simulink model "DataPath"  (R2025a)
settings: Solver=FixedStepAuto  StartTime=0  StopTime=0.02  FixedStep=1e-7  RelTol=1e-3
undefined symbols (not defined in the file): Bit_1, Bit_2, Bit_3, Bit_4, Bit_5, Bit_6, Bit_7, Bit_8
libraries: simulink_extras x126, fl_lib x34, nesl_utility x18, simulink x2
(part 1 of 7)
settings Model: PacingRate=0.000010  Creator=Erys  LastModifiedBy=Erys
settings DebuggingCC: AlgebraicLoopMsg=none  ForceCombineOutputUpdateInSim=on

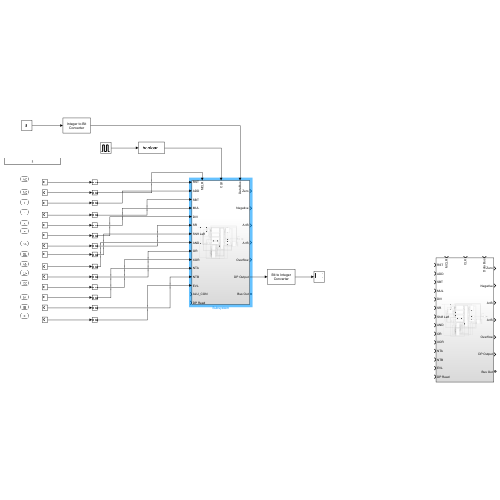
[thumbnail: Simulink's stored preview of the top-level diagram]
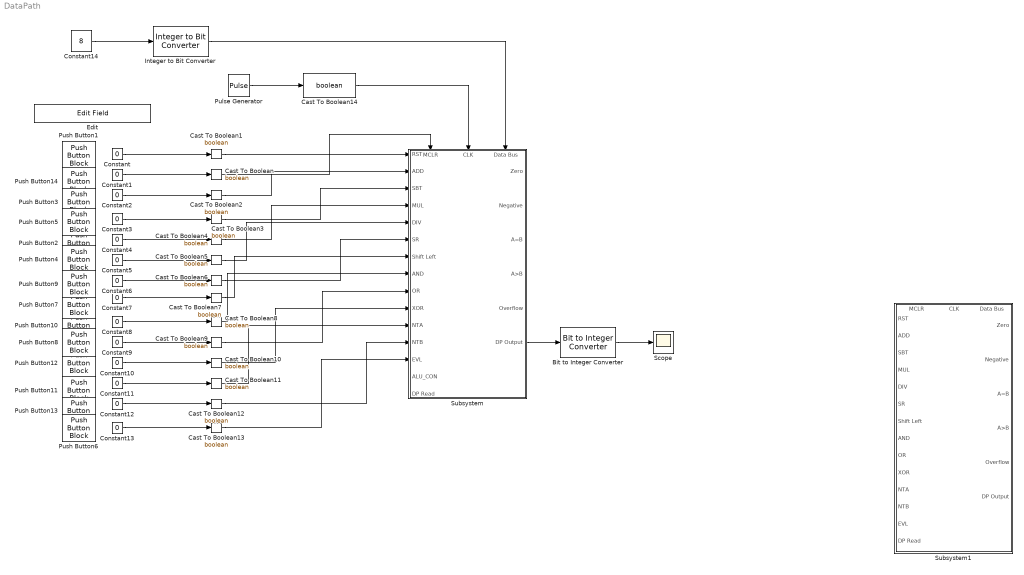
== system DataPath ==
  Bit to Integer Converter : simulink/Logic and Bit Operations/Bit to Integer Converter  nbits=8  bitOrder=MSB first  signedOutputValues=Unsigned  outDtype=Inherit via internal rule  outDtypeSigned=Inherit via internal rule
  Cast To Boolean{,1..14} (15 alike) : DataTypeConversion  OutDataTypeStr=boolean  SaturateOnIntegerOverflow=off  RndMeth=Floor
  Constant{,2..13} (13 alike) : Constant  Value=0
  Constant1 : Constant  Value=0  OutDataTypeStr=boolean
  Constant14 : Constant  Value=8
  Edit : EditField  LabelPosition=Hide  ShowInitialText=on  Alignment=Center
  Integer to Bit Converter : simulink/Logic and Bit Operations/Integer to Bit Converter  nbits=8  signedInputValues=Signed  bitOrder=MSB first  outDtype=Inherit via internal rule
  Pulse Generator : DiscretePulseGenerator  PulseType=Time based  Period=1e-6  PulseWidth=50
  Push Button1 : PushButtonBlock  ButtonText=AC  IconOnColor=[0.0, 0.39215686274509803, 0.0]  IconOffColor=[0.0, 1.0, 0.0]  OffValue=0.000000
  Push Button10 : PushButtonBlock  ButtonText=AND  IconOnColor=[0.0, 0.39215686274509803, 0.0]  IconOffColor=[0.0, 1.0, 0.0]  OffValue=0.000000
  Push Button11 : PushButtonBlock  ButtonText=!A  IconOnColor=[0.0, 0.39215686274509803, 0.0]  IconOffColor=[0.0, 1.0, 0.0]  OffValue=0.000000
  Push Button12 : PushButtonBlock  ButtonText=XOR  IconOnColor=[0.0, 0.39215686274509803, 0.0]  IconOffColor=[0.0, 1.0, 0.0]  OffValue=0.000000
  Push Button13 : PushButtonBlock  ButtonText=!B  IconOnColor=[0.0, 0.39215686274509803, 0.0]  IconOffColor=[0.0, 1.0, 0.0]  OffValue=0.000000
  Push Button14 : PushButtonBlock  ButtonText=MCLR  IconOnColor=[0.0, 0.39215686274509803, 0.0]  IconOffColor=[0.0, 1.0, 0.0]  OffValue=0.000000
  Push Button2 : PushButtonBlock  ButtonText=x  IconOnColor=[0.0, 0.39215686274509803, 0.0]  IconOffColor=[0.0, 1.0, 0.0]  OffValue=0.000000
  Push Button3 : PushButtonBlock  ButtonText=+  IconOnColor=[0.0, 0.39215686274509803, 0.0]  IconOffColor=[0.0, 1.0, 0.0]  OffValue=0.000000
  Push Button4 : PushButtonBlock  ButtonText=÷  IconOnColor=[0.0, 0.39215686274509803, 0.0]  IconOffColor=[0.0, 1.0, 0.0]  OffValue=0.000000
  Push Button5 : PushButtonBlock  ButtonText=-  IconOnColor=[0.0, 0.39215686274509803, 0.0]  IconOffColor=[0.0, 1.0, 0.0]  OffValue=0.000000
  Push Button6 : PushButtonBlock  ButtonText==  IconOnColor=[0.0, 0.39215686274509803, 0.0]  IconOffColor=[0.0, 1.0, 0.0]  OffValue=0.000000
  Push Button7 : PushButtonBlock  ButtonText=SL  IconOnColor=[0.0, 0.39215686274509803, 0.0]  IconOffColor=[0.0, 1.0, 0.0]  OffValue=0.000000
  Push Button8 : PushButtonBlock  ButtonText=OR  IconOnColor=[0.0, 0.39215686274509803, 0.0]  IconOffColor=[0.0, 1.0, 0.0]  OffValue=0.000000
  Push Button9 : PushButtonBlock  ButtonText=SR  IconOnColor=[0.0, 0.39215686274509803, 0.0]  IconOffColor=[0.0, 1.0, 0.0]  OffValue=0.000000
  Scope : Scope
      settings: ActiveDisplayYMinimum=-1.9999999999999996  ActiveDisplayYMaximum=18
  Subsystem : Subsystem
      settings: PortSchema="{\"entries\":[{\"content\":{\"sides\":[{\"content\":{\"connectorIds\":[\"In1\",\"In2\",\"In3\",\"In4\",\"In5\",\"In6\",\"In7\",\"In8\",\"In9\",\"In10\",\"In11\",\"In12\",\"In13\",\"In14\",\"In15\"]},\"type\":\"ConnectorPlacement.EquallySpacedRectSide\",\"uuid\":\"500cbc3b-e28d-47d3-99fc-6c714bf2f9c7\"},{\"content\":{\"connectorIds\":[\"Out1\",\"Out2\",\"Out3\",\"Out4\",\"Out5\",\"Out6\",\"RConn1\"],\"side\":\"RIGHT\"},\"type\":\"ConnectorPlacement.EquallySpacedRectSide\",\"uuid\":\"5d28cb21-17c3-47ed-8e1f-27c0d1cd1a3c\"},{\"content\":{\"connectorIds\":[\"In16\",\"In17\",\"In18\"],\"side\":\"TOP\"},\"type\":\"ConnectorPlacement.EquallySpacedRectSide\",\"uuid\":\"904f1374-4275-4bb1-a3cb-c22725edf960\"},{\"content\":{\"side\":\"BOTTOM\"},\"type\":\"ConnectorPlacement.EquallySpacedRectSide\",\"uuid\":\"1d94aa30-5d0f-4b17-8ccb-c29f6c482f2b\"}]},\"type\":\"ConnectorPlacement.EquallySpacedConnector\",\"uuid\":\"7b6858cb-ce34-402a-a17d-f8242b3d3948\"}],\"packageUris\":[\"http://schema.mathworks.com/mf0/Connector/R2020b\"],\"version\":\"1.0\"}"
  Subsystem1 : Subsystem
      settings: PortSchema="{\"entries\":[{\"content\":{\"sides\":[{\"content\":{\"connectorIds\":[\"In1\",\"In2\",\"In3\",\"In4\",\"In5\",\"In6\",\"In7\",\"In8\",\"In9\",\"In10\",\"In11\",\"In12\",\"In13\",\"In14\"]},\"type\":\"ConnectorPlacement.EquallySpacedRectSide\",\"uuid\":\"500cbc3b-e28d-47d3-99fc-6c714bf2f9c7\"},{\"content\":{\"connectorIds\":[\"Out1\",\"Out2\",\"Out3\",\"Out4\",\"Out5\",\"Out6\",\"RConn1\"],\"side\":\"RIGHT\"},\"type\":\"ConnectorPlacement.EquallySpacedRectSide\",\"uuid\":\"5d28cb21-17c3-47ed-8e1f-27c0d1cd1a3c\"},{\"content\":{\"connectorIds\":[\"In15\",\"In16\",\"In17\"],\"side\":\"TOP\"},\"type\":\"ConnectorPlacement.EquallySpacedRectSide\",\"uuid\":\"904f1374-4275-4bb1-a3cb-c22725edf960\"},{\"content\":{\"side\":\"BOTTOM\"},\"type\":\"ConnectorPlacement.EquallySpacedRectSide\",\"uuid\":\"1d94aa30-5d0f-4b17-8ccb-c29f6c482f2b\"}]},\"type\":\"ConnectorPlacement.EquallySpacedConnector\",\"uuid\":\"7b6858cb-ce34-402a-a17d-f8242b3d3948\"}],\"packageUris\":[\"http://schema.mathworks.com/mf0/Connector/R2020b\"],\"version\":\"1.0\"}"
  wires:
  Constant14/1 -> Integer to Bit Converter/1
  Constant4/1 -> Cast To Boolean4/1
  Constant5/1 -> Cast To Boolean5/1
  Constant3/1 -> Cast To Boolean3/1
  Integer to Bit Converter/1 -> Subsystem/18(Data Bus)
  Constant/1 -> Cast To Boolean1/1
  Constant1/1 -> Cast To Boolean/1
  Constant2/1 -> Cast To Boolean2/1
  Constant6/1 -> Cast To Boolean6/1
  Constant7/1 -> Cast To Boolean7/1
  Constant8/1 -> Cast To Boolean8/1
  Constant9/1 -> Cast To Boolean9/1
  Constant10/1 -> Cast To Boolean10/1
  Constant11/1 -> Cast To Boolean11/1
  Constant12/1 -> Cast To Boolean12/1
  Constant13/1 -> Cast To Boolean13/1
  Pulse Generator/1 -> Cast To Boolean14/1
  Cast To Boolean1/1 -> Subsystem/1(RST)
  Cast To Boolean/1 -> Subsystem/16(MCLR)
  Cast To Boolean2/1 -> Subsystem/2(ADD)
  Cast To Boolean3/1 -> Subsystem/3(SBT)
  Cast To Boolean4/1 -> Subsystem/4(MUL)
  Cast To Boolean5/1 -> Subsystem/5(DIV)
  Cast To Boolean6/1 -> Subsystem/6(SR)
  Cast To Boolean7/1 -> Subsystem/7(Shift Left)
  Cast To Boolean8/1 -> Subsystem/8(AND)
  Cast To Boolean9/1 -> Subsystem/9(OR)
  Cast To Boolean10/1 -> Subsystem/10(XOR)
  Cast To Boolean11/1 -> Subsystem/11(NTA)
  Cast To Boolean12/1 -> Subsystem/12(NTB)
  Cast To Boolean13/1 -> Subsystem/13(EVL)
  Subsystem/6(DP Output) -> Bit to Integer Converter/1
  Bit to Integer Converter/1 -> Scope/1
  Cast To Boolean14/1 -> Subsystem/17(CLK)

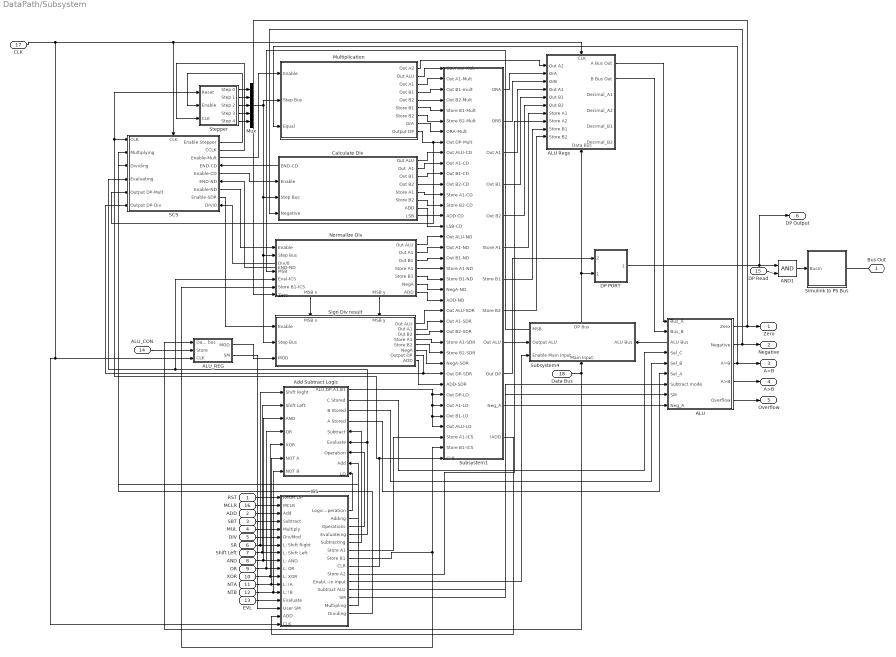
== system DataPath/Subsystem ==
  RST : Inport
  ADD : Inport  Port=2
  SBT : Inport  Port=3
  MUL : Inport  Port=4
  DIV : Inport  Port=5
  SR : Inport  Port=6
  Shift Left : Inport  Port=7
  AND : Inport  Port=8
  OR : Inport  Port=9
  XOR : Inport  Port=10
  NTA : Inport  Port=11
  NTB : Inport  Port=12
  EVL : Inport  Port=13
  ALU_CON : Inport  Port=14
  DP Read : Inport  Port=15
  MCLR : Inport  Port=16  OutDataTypeStr=boolean
  CLK : Inport  Port=17  OutDataTypeStr=boolean
  Data Bus : Inport  Port=18
  ALU : Subsystem
      settings: PortSchema="{\"entries\":[{\"content\":{\"sides\":[{\"content\":{\"connectorIds\":[\"In1\",\"In2\",\"Out6\",\"In3\",\"In4\",\"In5\",\"In6\",\"In7\",\"In8\"]},\"type\":\"ConnectorPlacement.EquallySpacedRectSide\",\"uuid\":\"c37a7539-9d16-4848-9066-29ecf491d7da\"},{\"content\":{\"connectorIds\":[\"Out1\",\"Out2\",\"Out3\",\"Out4\",\"Out5\"],\"side\":\"RIGHT\"},\"type\":\"ConnectorPlacement.EquallySpacedRectSide\",\"uuid\":\"a0e4cd93-9d4f-4763-9532-ee9322d920da\"},{\"content\":{\"side\":\"TOP\"},\"type\":\"ConnectorPlacement.EquallySpacedRectSide\",\"uuid\":\"186aeace-b60a-4a73-952e-f0bee95a6888\"}]},\"type\":\"ConnectorPlacement.EquallySpacedConnector\",\"uuid\":\"47b774ea-3904-45d1-ac98-1d3dfdc91dee\"}],\"packageUris\":[\"http://schema.mathworks.com/mf0/Connector/R2020b\"],\"version\":\"1.0\"}"
  ALU Regs : Subsystem
      settings: PortSchema="{\"entries\":[{\"content\":{\"sides\":[{\"content\":{\"connectorIds\":[\"In1\",\"In2\",\"In3\",\"In4\",\"In5\",\"In6\",\"In7\",\"In8\",\"In9\",\"In10\"]},\"type\":\"ConnectorPlacement.EquallySpacedRectSide\",\"uuid\":\"f897ceb0-c9b9-489e-8b32-2eb573f12d1a\"},{\"content\":{\"connectorIds\":[\"Out1\",\"Out2\",\"Out3\",\"Out4\",\"Out5\",\"Out6\"],\"side\":\"RIGHT\"},\"type\":\"ConnectorPlacement.EquallySpacedRectSide\",\"uuid\":\"50fe41fa-7ee3-4a8d-a06d-fa2133f944ed\"},{\"content\":{\"connectorIds\":[\"In11\"],\"side\":\"TOP\"},\"type\":\"ConnectorPlacement.EquallySpacedRectSide\",\"uuid\":\"9386cea2-fe71-481a-887c-1138907670aa\"},{\"content\":{\"connectorIds\":[\"In12\"],\"side\":\"BOTTOM\"},\"type\":\"ConnectorPlacement.EquallySpacedRectSide\",\"uuid\":\"2c9e15c6-049a-46aa-8a1e-0778ad228e2c\"}]},\"type\":\"ConnectorPlacement.EquallySpacedConnector\",\"uuid\":\"51e3a67b-2c64-426e-a2d7-da64166e8617\"}],\"packageUris\":[\"http://schema.mathworks.com/mf0/Connector/R2020b\"],\"version\":\"1.0\"}"
  ALU_REG : Subsystem
  AND1 : Logic  IconShape=distinctive  AllPortsSameDT=off  OutDataTypeStr=boolean
  Add Subtract Logic : Subsystem
      settings: PortSchema="{\"entries\":[{\"content\":{\"sides\":[{\"content\":{\"connectorIds\":[\"In1\",\"In2\",\"In3\",\"In4\",\"In5\",\"In6\",\"In7\"]},\"type\":\"ConnectorPlacement.EquallySpacedRectSide\",\"uuid\":\"155e8539-7b07-4c7c-9d9a-97cd4ac10054\"},{\"content\":{\"connectorIds\":[\"Out1\",\"Out2\",\"Out3\",\"Out4\",\"In8\",\"In9\",\"In10\",\"In11\",\"In12\"],\"side\":\"RIGHT\"},\"type\":\"ConnectorPlacement.EquallySpacedRectSide\",\"uuid\":\"e444004c-3fa4-46de-94bb-9c3dc8287e68\"},{\"content\":{\"side\":\"TOP\"},\"type\":\"ConnectorPlacement.EquallySpacedRectSide\",\"uuid\":\"07fd3642-a6d7-4398-b7f9-f213a05a7aff\"}]},\"type\":\"ConnectorPlacement.EquallySpacedConnector\",\"uuid\":\"401fffe2-fef7-4730-8c52-e9531038c85b\"}],\"packageUris\":[\"http://schema.mathworks.com/mf0/Connector/R2020b\"],\"version\":\"1.0\"}"
  Calculate Div : Subsystem
      settings: PortSchema="{\"entries\":[{\"content\":{\"sides\":[{\"content\":{\"connectorIds\":[\"Out9\",\"In1\",\"In2\",\"In3\"]},\"type\":\"ConnectorPlacement.EquallySpacedRectSide\",\"uuid\":\"248e61db-650f-41be-afeb-960a1b0fa547\"},{\"content\":{\"connectorIds\":[\"Out1\",\"Out2\",\"Out3\",\"Out4\",\"Out5\",\"Out6\",\"Out7\",\"Out8\"],\"side\":\"RIGHT\"},\"type\":\"ConnectorPlacement.EquallySpacedRectSide\",\"uuid\":\"a5a9d453-5aa0-49ce-8cbc-1e6a6fbe953d\"},{\"content\":{\"side\":\"TOP\"},\"type\":\"ConnectorPlacement.EquallySpacedRectSide\",\"uuid\":\"161ea693-d847-495c-b99e-fc66d877945e\"}]},\"type\":\"ConnectorPlacement.EquallySpacedConnector\",\"uuid\":\"e6ca75ed-542b-4a47-8d6b-6b616e1ea101\"}],\"packageUris\":[\"http://schema.mathworks.com/mf0/Connector/R2020b\"],\"version\":\"1.0\"}"
  DP PORT : Subsystem
  ICS : Subsystem
  Multiplication : Subsystem
  Mux : Mux  Inputs=5
  Normalize Div : Subsystem
      settings: PortSchema="{\"entries\":[{\"content\":{\"sides\":[{\"content\":{\"connectorIds\":[\"Out10\",\"In1\",\"In2\",\"Out11\",\"In3\",\"In4\",\"In5\",\"In6\"]},\"type\":\"ConnectorPlacement.EquallySpacedRectSide\",\"uuid\":\"3bf65de4-a84e-43af-85cb-ba419936807e\"},{\"content\":{\"connectorIds\":[\"Out1\",\"Out2\",\"Out3\",\"Out4\",\"Out5\",\"Out6\",\"Out7\"],\"side\":\"RIGHT\"},\"type\":\"ConnectorPlacement.EquallySpacedRectSide\",\"uuid\":\"49151b5f-73cb-49db-8fd7-1652ca273db5\"},{\"content\":{\"side\":\"TOP\"},\"type\":\"ConnectorPlacement.EquallySpacedRectSide\",\"uuid\":\"58143683-5a5d-47e2-b921-db5f028b3f5b\"},{\"content\":{\"connectorIds\":[\"Out8\",\"Out9\"],\"side\":\"BOTTOM\"},\"type\":\"ConnectorPlacement.EquallySpacedRectSide\",\"uuid\":\"3e5cf15a-3bf5-42b9-8752-baa0123e7179\"}]},\"type\":\"ConnectorPlacement.EquallySpacedConnector\",\"uuid\":\"daef8ab5-bc49-4af8-b635-2b796b1e5932\"}],\"packageUris\":[\"http://schema.mathworks.com/mf0/Connector/R2020b\"],\"version\":\"1.0\"}"
  SCS : Subsystem
      settings: PortSchema="{\"entries\":[{\"content\":{\"sides\":[{\"content\":{\"connectorIds\":[\"In1\",\"In2\",\"In3\",\"In4\",\"In5\",\"In6\"]},\"type\":\"ConnectorPlacement.EquallySpacedRectSide\",\"uuid\":\"5f827d29-1953-485f-9672-5b30f3e9777e\"},{\"content\":{\"connectorIds\":[\"Out1\",\"Out2\",\"Out3\",\"In8\",\"Out4\",\"In9\",\"Out5\",\"Out6\",\"In10\"],\"side\":\"RIGHT\"},\"type\":\"ConnectorPlacement.EquallySpacedRectSide\",\"uuid\":\"f4b83631-e908-4486-8992-7d28022d8f8a\"},{\"content\":{\"connectorIds\":[\"In7\"],\"side\":\"TOP\"},\"type\":\"ConnectorPlacement.EquallySpacedRectSide\",\"uuid\":\"92fa476f-0825-43c4-abf8-7a9cce9eadb6\"}]},\"type\":\"ConnectorPlacement.EquallySpacedConnector\",\"uuid\":\"7f47888f-0f87-43c3-bf1c-119855c5fec8\"}],\"packageUris\":[\"http://schema.mathworks.com/mf0/Connector/R2020b\"],\"version\":\"1.0\"}"
  Sign Div result : Subsystem
      settings: PortSchema="{\"entries\":[{\"content\":{\"sides\":[{\"content\":{\"connectorIds\":[\"In1\",\"In2\",\"In3\"]},\"type\":\"ConnectorPlacement.EquallySpacedRectSide\",\"uuid\":\"f5bc0604-c60b-487e-b7f2-96d42dc1b3a0\"},{\"content\":{\"connectorIds\":[\"Out1\",\"Out2\",\"Out3\",\"Out4\",\"Out5\",\"Out6\",\"Out7\",\"Out8\"],\"side\":\"RIGHT\"},\"type\":\"ConnectorPlacement.EquallySpacedRectSide\",\"uuid\":\"50d41b4c-a33b-4e34-b751-18ded5b2cb1e\"},{\"content\":{\"connectorIds\":[\"In4\",\"In5\"],\"side\":\"TOP\"},\"type\":\"ConnectorPlacement.EquallySpacedRectSide\",\"uuid\":\"1ba562d7-8709-4333-a841-74571fdc4e92\"}]},\"type\":\"ConnectorPlacement.EquallySpacedConnector\",\"uuid\":\"8253a047-369e-44b5-9bb6-13f033f299b7\"}],\"packageUris\":[\"http://schema.mathworks.com/mf0/Connector/R2020b\"],\"version\":\"1.0\"}"
  Simulink to PS Bus : Subsystem
  Stepper : Subsystem
  Subsystem1 : Subsystem
  Subsystem4 : Subsystem
      settings: PortSchema="{\"entries\":[{\"content\":{\"sides\":[{\"content\":{\"connectorIds\":[\"Out2\"]},\"type\":\"ConnectorPlacement.EquallySpacedRectSide\",\"uuid\":\"d8595652-6905-4cc2-aa18-713ce57c3b65\"},{\"content\":{\"connectorIds\":[\"In4\"],\"side\":\"RIGHT\"},\"type\":\"ConnectorPlacement.EquallySpacedRectSide\",\"uuid\":\"5abc3ebd-ff8c-460a-ade3-5894559f8820\"},{\"content\":{\"connectorIds\":[\"Out1\",\"In1\",\"In2\"],\"side\":\"TOP\"},\"type\":\"ConnectorPlacement.EquallySpacedRectSide\",\"uuid\":\"929f6aeb-a855-409a-8e7c-28fb07fb21dc\"},{\"content\":{\"connectorIds\":[\"In3\"],\"side\":\"BOTTOM\"},\"type\":\"ConnectorPlacement.EquallySpacedRectSide\",\"uuid\":\"480c7dc4-4298-475d-8e28-71ecbd723b86\"}]},\"type\":\"ConnectorPlacement.EquallySpacedConnector\",\"uuid\":\"31897c44-8fce-467c-9d36-164830a373ff\"}],\"packageUris\":[\"http://schema.mathworks.com/mf0/Connector/R2020b\"],\"version\":\"1.0\"}"
  Bus Out : PMIOPort  Side=Right
  Zero : Outport
  Negative : Outport  Port=2
  A=B : Outport  Port=3
  A>B : Outport  Port=4
  Overflow : Outport  Port=5
  DP Output : Outport  Port=6
  wires:
  Stepper/1(Step 0) -> Mux/1
  Stepper/2(Step 1) -> Mux/2
  Stepper/5(Step 4) -> Mux/5
  Stepper/4(Step 3) -> Mux/4
  Stepper/3(Step 2) -> Mux/3
  Normalize Div/8(MSB x) -> Sign Div result/4(MSB x)
  Normalize Div/9(MSB y) -> Sign Div result/5(MSB y)
  Multiplication/2(Out ALU) -> Subsystem1/1(Out ALU-Mult)
  Multiplication/3(Out A1) -> Subsystem1/2(Out A1-Mult)
  Multiplication/4(Out B1) -> Subsystem1/3(Out B1-mult)
  Multiplication/5(Out B2) -> Subsystem1/4(Out B2-Mult)
  Multiplication/6(Store B1) -> Subsystem1/5(Store B1-Mult)
  Multiplication/7(Store B2) -> Subsystem1/6(Store B2-Mult)
  Multiplication/8(OrA) -> Subsystem1/7(ORA-Mult)
  Multiplication/9(Output DP) -> SCS/5(Output DP-Mult), Subsystem1/8(Out DP-Mult)
  Calculate Div/1(Out ALU) -> Subsystem1/9(Out ALU-CD)
  Calculate Div/2(Out  A1) -> Subsystem1/10(Out A1-CD)
  Calculate Div/5(Store A1) -> Subsystem1/13(Store A1-CD)
  Calculate Div/6(Store B2) -> Subsystem1/14(Store B2-CD)
  Calculate Div/7(ADD) -> Subsystem1/15(ADD CD)
  Calculate Div/8(LSB) -> Subsystem1/16(LSB-CD)
  Normalize Div/1(Out ALU) -> Subsystem1/17(Out ALU-ND)
  Normalize Div/2(Out A1) -> Subsystem1/18(Out A1-ND)
  Normalize Div/3(Out B1) -> Subsystem1/19(Out B1-ND)
  Normalize Div/4(Store A1) -> Subsystem1/20(Store A1-ND)
  Normalize Div/5(Store B1) -> Subsystem1/21(Store B1-ND)
  Normalize Div/6(NegA) -> Subsystem1/22(NegA-ND)
  Normalize Div/7(ADD) -> Subsystem1/23(ADD-ND)
  Sign Div result/1(Out ALU) -> Subsystem1/24(Out ALU-SDR)
  Sign Div result/2(Out A1) -> Subsystem1/25(Out A1-SDR)
  Sign Div result/3(Out B2) -> Subsystem1/26(Out B2-SDR)
  Sign Div result/4(Store A1) -> Subsystem1/27(Store A1-SDR)
  Sign Div result/5(Store B2) -> Subsystem1/28(Store B2-SDR)
  Sign Div result/6(NegA) -> Subsystem1/29(NegA-SDR)
  Sign Div result/7(Output DP) -> SCS/6(Output DP-Div), Subsystem1/30(Out DP-SDR)
  Add Subtract Logic/1(ALU,DP,A1,B1) -> Subsystem1/32(Out DP-LO), Subsystem1/33(Out A1-LO), Subsystem1/34(Out B1-LO), Subsystem1/35(Out ALU-LO)
  ICS/6(Store A1) -> Subsystem1/36(Store A1-ICS)
  ICS/7(Store B1) -> Subsystem1/37(Store B1-ICS), Normalize Div/5(Store B1-ICS)
  ICS/8(CLR) -> Subsystem1/38(CLR), SCS/1(CLR), Stepper/1(Reset)
  SCS/3(Enable-Mult) -> Multiplication/1(Enable)
  Calculate Div/9(END-CD) -> SCS/8(END-CD)
  SCS/4(Enable-CD) -> Calculate Div/1(Enable)
  Normalize Div/10(END-ND) -> SCS/9(END-ND)
  SCS/5(Enable-ND) -> Normalize Div/1(Enable)
  SCS/6(Enable-SDR) -> Sign Div result/1(Enable)
  Mux/1 -> Calculate Div/2(Step Bus), Sign Div result/2(Step Bus), Normalize Div/2(Step Bus), Multiplication/2(Step Bus)
  SCS/1(Enable Stepper) -> Stepper/2(Enable)
  SCS/2(CCLK) -> Stepper/3(CLK)
  Normalize Div/11(Div/0) -> SCS/10(DIV/0)
  ICS/10(Enable main input) -> Subsystem4/2(Enable Main Input)
  Subsystem1/9(Out ALU) -> Subsystem4/1(Output ALU)
  Subsystem1/10(Out DP) -> DP PORT/2(Enable)
  ALU/6(ALU Bus) -> Subsystem4/3(ALU Bus)
  Subsystem4/2(DP Bus) -> ALU Regs/12(Data Bus), DP PORT/1(DP Bus)
  Subsystem1/3(Out A1) -> ALU Regs/4(Out A1)
  Subsystem1/4(Out B1) -> ALU Regs/5(Out B1)
  Subsystem1/5(Out B2) -> ALU Regs/6(Out B2)
  Subsystem1/6(Store A1) -> ALU Regs/7(Store A1)
  Subsystem1/8(Store B2) -> ALU Regs/10(Store B2)
  Subsystem1/11(Neg_A) -> ALU/8(Neg_A)
  Multiplication/1(Out A2) -> ALU Regs/1(Out A2)
  Add Subtract Logic/2(C Stored) -> ALU/3(Sel_C)
  Add Subtract Logic/3(B Stored) -> ALU/4(Sel_B)
  Add Subtract Logic/4(A Stored) -> ALU/5(Sel_A)
  ALU Regs/1(A Bus Out) -> ALU/1(Bus_A)
  ALU Regs/2(B Bus Out) -> ALU/2(Bus_B)
  ICS/9(Store A2) -> ALU Regs/8(Store A2)
  Subsystem1/7(Store B1) -> ALU Regs/9(Store B1)
  ALU/2(Negative) -> Negative/1, Calculate Div/3(Negative)
  ALU/1(Zero) -> Zero/1, Normalize Div/6(Zero)
  ALU/3(A=B) -> A=B/1, Multiplication/3(Equal)
  ALU/4(A>B) -> A>B/1
  RST/1 -> ICS/1(Reset DP)
  MCLR/1 -> ICS/2(MCLR)
  ADD/1 -> ICS/3(Add)
  SBT/1 -> ICS/4(Subtract)
  MUL/1 -> ICS/5(Multiply)
  DIV/1 -> ICS/6(Div/Mod)
  SR/1 -> Add Subtract Logic/1(Shift Right), ICS/7(L: Shift Right)
  Shift Left/1 -> Add Subtract Logic/2(Shift Left), ICS/8(L: Shift Left)
  AND/1 -> ICS/9(L: AND), Add Subtract Logic/3(AND)
  OR/1 -> Add Subtract Logic/4(OR), ICS/10(L: OR)
  XOR/1 -> Add Subtract Logic/5(XOR), ICS/11(L: XOR)
  NTA/1 -> Add Subtract Logic/6(NOT A), ICS/12(L: !A)
  NTB/1 -> Add Subtract Logic/7(NOT B), ICS/13(L: !B)
  EVL/1 -> ICS/14(Evaluate)
  ALU_REG/2(SM) -> ICS/15(User SM)
  Subsystem1/12("!ADD ") -> ICS/16(ADD)
  ICS/1(Logic Operation) -> Add Subtract Logic/12(LO)
  ICS/2(Adding) -> Add Subtract Logic/11(Add)
  ICS/3(Operations) -> Add Subtract Logic/10(Operation)
  ICS/4(Evaluateing) -> Add Subtract Logic/9(Evaluate), SCS/4(Evaluating), Normalize Div/4(Eval-ICS)
  ICS/5(Subtracting) -> Add Subtract Logic/8(Subtract)
  ICS/11(Subtract ALU) -> ALU/6(Subtract mode)
  ICS/12(SM) -> ALU/7(SM)
  ICS/13(Multipling) -> SCS/2(Multiplying)
  ICS/14(Dividing) -> SCS/3(Dividing)
  CLK/1 -> SCS/7(CLK), ALU Regs/11(CLK), ALU_REG/3(CLK), ICS/17(CLK)
  ALU_CON/1 -> ALU_REG/2(Store)
  DP PORT/1(DP Output) -> DP Output/1, AND1/1
  Subsystem4/1(MSB) -> Normalize Div/3(MSB)
  Data Bus/1 -> Subsystem4/4(Main Input), ALU_REG/1(Data bus)
  Subsystem1/1(ORA) -> ALU Regs/2(OrA)
  Subsystem1/2(ORB) -> ALU Regs/3(OrB)
  Calculate Div/3(Out B1) -> Subsystem1/11(Out B1-CD)
  Calculate Div/4(Out B2) -> Subsystem1/12(Out B2-CD)
  Sign Div result/8(ADD) -> Subsystem1/31(ADD-SDR)
  ALU/5(Overflow) -> Overflow/1
  ALU_REG/1(MOD) -> Sign Div result/3(MOD)
  AND1/1 -> Simulink to PS Bus/1(BusIn)
  DP Read/1 -> AND1/2
  connections:
  Bus Out/RConn1 -- Simulink to PS Bus/RConn1

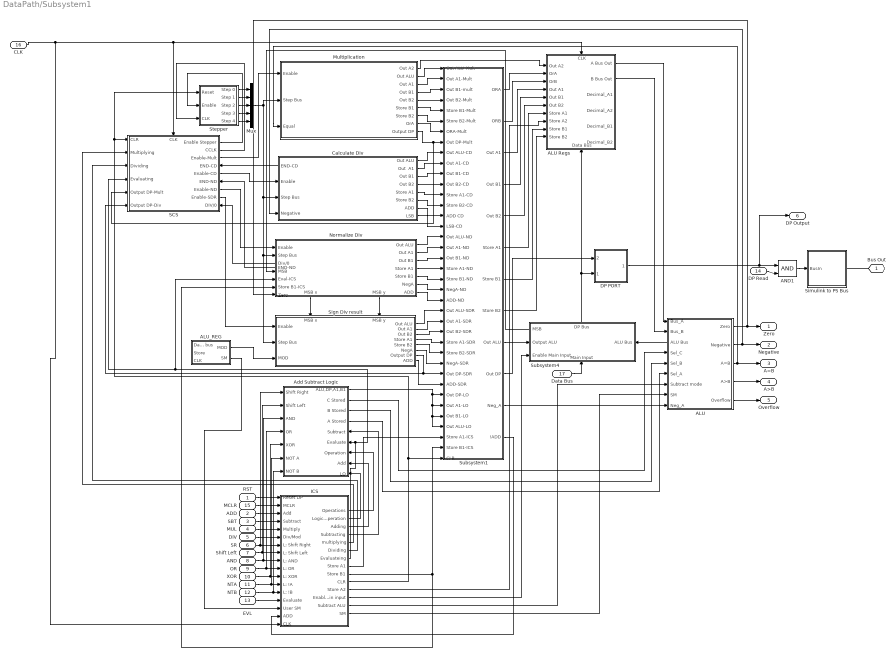
== system DataPath/Subsystem1 ==
  RST : Inport
  ADD : Inport  Port=2
  SBT : Inport  Port=3
  MUL : Inport  Port=4
  DIV : Inport  Port=5
  SR : Inport  Port=6
  Shift Left : Inport  Port=7
  AND : Inport  Port=8
  OR : Inport  Port=9
  XOR : Inport  Port=10
  NTA : Inport  Port=11
  NTB : Inport  Port=12
  EVL : Inport  Port=13
  DP Read : Inport  Port=14
  MCLR : Inport  Port=15  OutDataTypeStr=boolean
  CLK : Inport  Port=16  OutDataTypeStr=boolean
  Data Bus : Inport  Port=17
  ALU : Subsystem
      settings: PortSchema="{\"entries\":[{\"content\":{\"sides\":[{\"content\":{\"connectorIds\":[\"In1\",\"In2\",\"Out6\",\"In3\",\"In4\",\"In5\",\"In6\",\"In7\",\"In8\"]},\"type\":\"ConnectorPlacement.EquallySpacedRectSide\",\"uuid\":\"c37a7539-9d16-4848-9066-29ecf491d7da\"},{\"content\":{\"connectorIds\":[\"Out1\",\"Out2\",\"Out3\",\"Out4\",\"Out5\"],\"side\":\"RIGHT\"},\"type\":\"ConnectorPlacement.EquallySpacedRectSide\",\"uuid\":\"a0e4cd93-9d4f-4763-9532-ee9322d920da\"},{\"content\":{\"side\":\"TOP\"},\"type\":\"ConnectorPlacement.EquallySpacedRectSide\",\"uuid\":\"186aeace-b60a-4a73-952e-f0bee95a6888\"}]},\"type\":\"ConnectorPlacement.EquallySpacedConnector\",\"uuid\":\"47b774ea-3904-45d1-ac98-1d3dfdc91dee\"}],\"packageUris\":[\"http://schema.mathworks.com/mf0/Connector/R2020b\"],\"version\":\"1.0\"}"
  ALU Regs : Subsystem
      settings: PortSchema="{\"entries\":[{\"content\":{\"sides\":[{\"content\":{\"connectorIds\":[\"In1\",\"In2\",\"In3\",\"In4\",\"In5\",\"In6\",\"In7\",\"In8\",\"In9\",\"In10\"]},\"type\":\"ConnectorPlacement.EquallySpacedRectSide\",\"uuid\":\"f897ceb0-c9b9-489e-8b32-2eb573f12d1a\"},{\"content\":{\"connectorIds\":[\"Out1\",\"Out2\",\"Out3\",\"Out4\",\"Out5\",\"Out6\"],\"side\":\"RIGHT\"},\"type\":\"ConnectorPlacement.EquallySpacedRectSide\",\"uuid\":\"50fe41fa-7ee3-4a8d-a06d-fa2133f944ed\"},{\"content\":{\"connectorIds\":[\"In11\"],\"side\":\"TOP\"},\"type\":\"ConnectorPlacement.EquallySpacedRectSide\",\"uuid\":\"9386cea2-fe71-481a-887c-1138907670aa\"},{\"content\":{\"connectorIds\":[\"In12\"],\"side\":\"BOTTOM\"},\"type\":\"ConnectorPlacement.EquallySpacedRectSide\",\"uuid\":\"2c9e15c6-049a-46aa-8a1e-0778ad228e2c\"}]},\"type\":\"ConnectorPlacement.EquallySpacedConnector\",\"uuid\":\"51e3a67b-2c64-426e-a2d7-da64166e8617\"}],\"packageUris\":[\"http://schema.mathworks.com/mf0/Connector/R2020b\"],\"version\":\"1.0\"}"
  ALU_REG : Subsystem
  AND1 : Logic  IconShape=distinctive  AllPortsSameDT=off  OutDataTypeStr=boolean
  Add Subtract Logic : Subsystem
      settings: PortSchema="{\"entries\":[{\"content\":{\"sides\":[{\"content\":{\"connectorIds\":[\"In1\",\"In2\",\"In3\",\"In4\",\"In5\",\"In6\",\"In7\"]},\"type\":\"ConnectorPlacement.EquallySpacedRectSide\",\"uuid\":\"155e8539-7b07-4c7c-9d9a-97cd4ac10054\"},{\"content\":{\"connectorIds\":[\"Out1\",\"Out2\",\"Out3\",\"Out4\",\"In8\",\"In9\",\"In10\",\"In11\",\"In12\"],\"side\":\"RIGHT\"},\"type\":\"ConnectorPlacement.EquallySpacedRectSide\",\"uuid\":\"e444004c-3fa4-46de-94bb-9c3dc8287e68\"},{\"content\":{\"side\":\"TOP\"},\"type\":\"ConnectorPlacement.EquallySpacedRectSide\",\"uuid\":\"07fd3642-a6d7-4398-b7f9-f213a05a7aff\"}]},\"type\":\"ConnectorPlacement.EquallySpacedConnector\",\"uuid\":\"401fffe2-fef7-4730-8c52-e9531038c85b\"}],\"packageUris\":[\"http://schema.mathworks.com/mf0/Connector/R2020b\"],\"version\":\"1.0\"}"
  Calculate Div : Subsystem
      settings: PortSchema="{\"entries\":[{\"content\":{\"sides\":[{\"content\":{\"connectorIds\":[\"Out9\",\"In1\",\"In2\",\"In3\"]},\"type\":\"ConnectorPlacement.EquallySpacedRectSide\",\"uuid\":\"248e61db-650f-41be-afeb-960a1b0fa547\"},{\"content\":{\"connectorIds\":[\"Out1\",\"Out2\",\"Out3\",\"Out4\",\"Out5\",\"Out6\",\"Out7\",\"Out8\"],\"side\":\"RIGHT\"},\"type\":\"ConnectorPlacement.EquallySpacedRectSide\",\"uuid\":\"a5a9d453-5aa0-49ce-8cbc-1e6a6fbe953d\"},{\"content\":{\"side\":\"TOP\"},\"type\":\"ConnectorPlacement.EquallySpacedRectSide\",\"uuid\":\"161ea693-d847-495c-b99e-fc66d877945e\"}]},\"type\":\"ConnectorPlacement.EquallySpacedConnector\",\"uuid\":\"e6ca75ed-542b-4a47-8d6b-6b616e1ea101\"}],\"packageUris\":[\"http://schema.mathworks.com/mf0/Connector/R2020b\"],\"version\":\"1.0\"}"
  DP PORT : Subsystem
  ICS : Subsystem
  Multiplication : Subsystem
  Mux : Mux  Inputs=5
  Normalize Div : Subsystem
      settings: PortSchema="{\"entries\":[{\"content\":{\"sides\":[{\"content\":{\"connectorIds\":[\"Out10\",\"In1\",\"In2\",\"Out11\",\"In3\",\"In4\",\"In5\",\"In6\"]},\"type\":\"ConnectorPlacement.EquallySpacedRectSide\",\"uuid\":\"3bf65de4-a84e-43af-85cb-ba419936807e\"},{\"content\":{\"connectorIds\":[\"Out1\",\"Out2\",\"Out3\",\"Out4\",\"Out5\",\"Out6\",\"Out7\"],\"side\":\"RIGHT\"},\"type\":\"ConnectorPlacement.EquallySpacedRectSide\",\"uuid\":\"49151b5f-73cb-49db-8fd7-1652ca273db5\"},{\"content\":{\"side\":\"TOP\"},\"type\":\"ConnectorPlacement.EquallySpacedRectSide\",\"uuid\":\"58143683-5a5d-47e2-b921-db5f028b3f5b\"},{\"content\":{\"connectorIds\":[\"Out8\",\"Out9\"],\"side\":\"BOTTOM\"},\"type\":\"ConnectorPlacement.EquallySpacedRectSide\",\"uuid\":\"3e5cf15a-3bf5-42b9-8752-baa0123e7179\"}]},\"type\":\"ConnectorPlacement.EquallySpacedConnector\",\"uuid\":\"daef8ab5-bc49-4af8-b635-2b796b1e5932\"}],\"packageUris\":[\"http://schema.mathworks.com/mf0/Connector/R2020b\"],\"version\":\"1.0\"}"
  SCS : Subsystem
      settings: PortSchema="{\"entries\":[{\"content\":{\"sides\":[{\"content\":{\"connectorIds\":[\"In1\",\"In2\",\"In3\",\"In4\",\"In5\",\"In6\"]},\"type\":\"ConnectorPlacement.EquallySpacedRectSide\",\"uuid\":\"5f827d29-1953-485f-9672-5b30f3e9777e\"},{\"content\":{\"connectorIds\":[\"Out1\",\"Out2\",\"Out3\",\"In8\",\"Out4\",\"In9\",\"Out5\",\"Out6\",\"In10\"],\"side\":\"RIGHT\"},\"type\":\"ConnectorPlacement.EquallySpacedRectSide\",\"uuid\":\"f4b83631-e908-4486-8992-7d28022d8f8a\"},{\"content\":{\"connectorIds\":[\"In7\"],\"side\":\"TOP\"},\"type\":\"ConnectorPlacement.EquallySpacedRectSide\",\"uuid\":\"92fa476f-0825-43c4-abf8-7a9cce9eadb6\"}]},\"type\":\"ConnectorPlacement.EquallySpacedConnector\",\"uuid\":\"7f47888f-0f87-43c3-bf1c-119855c5fec8\"}],\"packageUris\":[\"http://schema.mathworks.com/mf0/Connector/R2020b\"],\"version\":\"1.0\"}"
  Sign Div result : Subsystem
      settings: PortSchema="{\"entries\":[{\"content\":{\"sides\":[{\"content\":{\"connectorIds\":[\"In1\",\"In2\",\"In3\"]},\"type\":\"ConnectorPlacement.EquallySpacedRectSide\",\"uuid\":\"f5bc0604-c60b-487e-b7f2-96d42dc1b3a0\"},{\"content\":{\"connectorIds\":[\"Out1\",\"Out2\",\"Out3\",\"Out4\",\"Out5\",\"Out6\",\"Out7\",\"Out8\"],\"side\":\"RIGHT\"},\"type\":\"ConnectorPlacement.EquallySpacedRectSide\",\"uuid\":\"50d41b4c-a33b-4e34-b751-18ded5b2cb1e\"},{\"content\":{\"connectorIds\":[\"In4\",\"In5\"],\"side\":\"TOP\"},\"type\":\"ConnectorPlacement.EquallySpacedRectSide\",\"uuid\":\"1ba562d7-8709-4333-a841-74571fdc4e92\"}]},\"type\":\"ConnectorPlacement.EquallySpacedConnector\",\"uuid\":\"8253a047-369e-44b5-9bb6-13f033f299b7\"}],\"packageUris\":[\"http://schema.mathworks.com/mf0/Connector/R2020b\"],\"version\":\"1.0\"}"
  Simulink to PS Bus : Subsystem
  Stepper : Subsystem
  Subsystem1 : Subsystem
  Subsystem4 : Subsystem
      settings: PortSchema="{\"entries\":[{\"content\":{\"sides\":[{\"content\":{\"connectorIds\":[\"Out2\"]},\"type\":\"ConnectorPlacement.EquallySpacedRectSide\",\"uuid\":\"d8595652-6905-4cc2-aa18-713ce57c3b65\"},{\"content\":{\"connectorIds\":[\"In4\"],\"side\":\"RIGHT\"},\"type\":\"ConnectorPlacement.EquallySpacedRectSide\",\"uuid\":\"5abc3ebd-ff8c-460a-ade3-5894559f8820\"},{\"content\":{\"connectorIds\":[\"Out1\",\"In1\",\"In2\"],\"side\":\"TOP\"},\"type\":\"ConnectorPlacement.EquallySpacedRectSide\",\"uuid\":\"929f6aeb-a855-409a-8e7c-28fb07fb21dc\"},{\"content\":{\"connectorIds\":[\"In3\"],\"side\":\"BOTTOM\"},\"type\":\"ConnectorPlacement.EquallySpacedRectSide\",\"uuid\":\"480c7dc4-4298-475d-8e28-71ecbd723b86\"}]},\"type\":\"ConnectorPlacement.EquallySpacedConnector\",\"uuid\":\"31897c44-8fce-467c-9d36-164830a373ff\"}],\"packageUris\":[\"http://schema.mathworks.com/mf0/Connector/R2020b\"],\"version\":\"1.0\"}"
  Bus Out : PMIOPort  Side=Right
  Zero : Outport
  Negative : Outport  Port=2
  A=B : Outport  Port=3
  A>B : Outport  Port=4
  Overflow : Outport  Port=5
  DP Output : Outport  Port=6
  wires:
  Stepper/1(Step 0) -> Mux/1
  Stepper/2(Step 1) -> Mux/2
  Stepper/5(Step 4) -> Mux/5
  Stepper/4(Step 3) -> Mux/4
  Stepper/3(Step 2) -> Mux/3
  Normalize Div/8(MSB x) -> Sign Div result/4(MSB x)
  Normalize Div/9(MSB y) -> Sign Div result/5(MSB y)
  Multiplication/2(Out ALU) -> Subsystem1/1(Out ALU-Mult)
  Multiplication/3(Out A1) -> Subsystem1/2(Out A1-Mult)
  Multiplication/4(Out B1) -> Subsystem1/3(Out B1-mult)
  Multiplication/5(Out B2) -> Subsystem1/4(Out B2-Mult)
  Multiplication/6(Store B1) -> Subsystem1/5(Store B1-Mult)
  Multiplication/7(Store B2) -> Subsystem1/6(Store B2-Mult)
  Multiplication/8(OrA) -> Subsystem1/7(ORA-Mult)
  Multiplication/9(Output DP) -> SCS/5(Output DP-Mult), Subsystem1/8(Out DP-Mult)
  Calculate Div/1(Out ALU) -> Subsystem1/9(Out ALU-CD)
  Calculate Div/2(Out  A1) -> Subsystem1/10(Out A1-CD)
  Calculate Div/5(Store A1) -> Subsystem1/13(Store A1-CD)
  Calculate Div/6(Store B2) -> Subsystem1/14(Store B2-CD)
  Calculate Div/7(ADD) -> Subsystem1/15(ADD CD)
  Calculate Div/8(LSB) -> Subsystem1/16(LSB-CD)
  Normalize Div/1(Out ALU) -> Subsystem1/17(Out ALU-ND)
  Normalize Div/2(Out A1) -> Subsystem1/18(Out A1-ND)
  Normalize Div/3(Out B1) -> Subsystem1/19(Out B1-ND)
  Normalize Div/4(Store A1) -> Subsystem1/20(Store A1-ND)
  Normalize Div/5(Store B1) -> Subsystem1/21(Store B1-ND)
  Normalize Div/6(NegA) -> Subsystem1/22(NegA-ND)
  Normalize Div/7(ADD) -> Subsystem1/23(ADD-ND)
  Sign Div result/1(Out ALU) -> Subsystem1/24(Out ALU-SDR)
  Sign Div result/2(Out A1) -> Subsystem1/25(Out A1-SDR)
  Sign Div result/3(Out B2) -> Subsystem1/26(Out B2-SDR)
  Sign Div result/4(Store A1) -> Subsystem1/27(Store A1-SDR)
  Sign Div result/5(Store B2) -> Subsystem1/28(Store B2-SDR)
  Sign Div result/6(NegA) -> Subsystem1/29(NegA-SDR)
  Sign Div result/7(Output DP) -> SCS/6(Output DP-Div), Subsystem1/30(Out DP-SDR)
  Add Subtract Logic/1(ALU,DP,A1,B1) -> Subsystem1/32(Out DP-LO), Subsystem1/33(Out A1-LO), Subsystem1/34(Out B1-LO), Subsystem1/35(Out ALU-LO)
  ICS/8(Store A1) -> Subsystem1/36(Store A1-ICS)
  ICS/9(Store B1) -> Subsystem1/37(Store B1-ICS), Normalize Div/5(Store B1-ICS)
  ICS/10(CLR) -> Subsystem1/38(CLR), SCS/1(CLR), Stepper/1(Reset)
  SCS/3(Enable-Mult) -> Multiplication/1(Enable)
  Calculate Div/9(END-CD) -> SCS/8(END-CD)
  SCS/4(Enable-CD) -> Calculate Div/1(Enable)
  Normalize Div/10(END-ND) -> SCS/9(END-ND)
  SCS/5(Enable-ND) -> Normalize Div/1(Enable)
  SCS/6(Enable-SDR) -> Sign Div result/1(Enable)
  Mux/1 -> Calculate Div/2(Step Bus), Sign Div result/2(Step Bus), Normalize Div/2(Step Bus), Multiplication/2(Step Bus)
  SCS/1(Enable Stepper) -> Stepper/2(Enable)
  SCS/2(CCLK) -> Stepper/3(CLK)
  Normalize Div/11(Div/0) -> SCS/10(DIV/0)
  ICS/12(Enable main input) -> Subsystem4/2(Enable Main Input)
  Subsystem1/9(Out ALU) -> Subsystem4/1(Output ALU)
  Subsystem1/10(Out DP) -> DP PORT/2(Enable)
  ALU/6(ALU Bus) -> Subsystem4/3(ALU Bus)
  Subsystem4/2(DP Bus) -> ALU Regs/12(Data Bus), DP PORT/1(DP Bus)
  Subsystem1/3(Out A1) -> ALU Regs/4(Out A1)
  Subsystem1/4(Out B1) -> ALU Regs/5(Out B1)
  Subsystem1/5(Out B2) -> ALU Regs/6(Out B2)
  Subsystem1/6(Store A1) -> ALU Regs/7(Store A1)
  Subsystem1/8(Store B2) -> ALU Regs/10(Store B2)
  Subsystem1/11(Neg_A) -> ALU/8(Neg_A)
  Multiplication/1(Out A2) -> ALU Regs/1(Out A2)
  Add Subtract Logic/2(C Stored) -> ALU/3(Sel_C)
  Add Subtract Logic/3(B Stored) -> ALU/4(Sel_B)
  Add Subtract Logic/4(A Stored) -> ALU/5(Sel_A)
  ALU Regs/1(A Bus Out) -> ALU/1(Bus_A)
  ALU Regs/2(B Bus Out) -> ALU/2(Bus_B)
  ICS/11(Store A2) -> ALU Regs/8(Store A2)
  Subsystem1/7(Store B1) -> ALU Regs/9(Store B1)
  ALU/2(Negative) -> Negative/1, Calculate Div/3(Negative)
  ALU/1(Zero) -> Zero/1, Normalize Div/6(Zero)
  ALU/3(A=B) -> A=B/1, Multiplication/3(Equal)
  ALU/4(A>B) -> A>B/1
  RST/1 -> ICS/1(Reset DP)
  MCLR/1 -> ICS/2(MCLR)
  ADD/1 -> ICS/3(Add)
  SBT/1 -> ICS/4(Subtract)
  MUL/1 -> ICS/5(Multiply)
  DIV/1 -> ICS/6(Div/Mod)
  SR/1 -> Add Subtract Logic/1(Shift Right), ICS/7(L: Shift Right)
  Shift Left/1 -> Add Subtract Logic/2(Shift Left), ICS/8(L: Shift Left)
  AND/1 -> ICS/9(L: AND), Add Subtract Logic/3(AND)
  OR/1 -> Add Subtract Logic/4(OR), ICS/10(L: OR)
  XOR/1 -> Add Subtract Logic/5(XOR), ICS/11(L: XOR)
  NTA/1 -> Add Subtract Logic/6(NOT A), ICS/12(L: !A)
  NTB/1 -> Add Subtract Logic/7(NOT B), ICS/13(L: !B)
  EVL/1 -> ICS/14(Evaluate)
  ALU_REG/2(SM) -> ICS/15(User SM)
  Subsystem1/12("!ADD ") -> ICS/16(ADD)
  ICS/2(Logic Operation) -> Add Subtract Logic/12(LO)
  ICS/3(Adding) -> Add Subtract Logic/11(Add)
  ICS/1(Operations) -> Add Subtract Logic/10(Operation)
  ICS/7(Evaluateing) -> SCS/4(Evaluating), Normalize Div/4(Eval-ICS), Add Subtract Logic/9(Evaluate)
  ICS/4(Subtracting) -> Add Subtract Logic/8(Subtract)
  ICS/13(Subtract ALU) -> ALU/6(Subtract mode)
  ICS/14(SM) -> ALU/7(SM)
  ICS/5("multiplying ") -> SCS/2(Multiplying)
  ICS/6(Dividing) -> SCS/3(Dividing)
  CLK/1 -> SCS/7(CLK), ALU Regs/11(CLK), ICS/17(CLK)
  DP PORT/1(DP Output) -> DP Output/1, AND1/1
  Subsystem4/1(MSB) -> Normalize Div/3(MSB)
  Data Bus/1 -> Subsystem4/4(Main Input)
  Subsystem1/1(ORA) -> ALU Regs/2(OrA)
  Subsystem1/2(ORB) -> ALU Regs/3(OrB)
  Calculate Div/3(Out B1) -> Subsystem1/11(Out B1-CD)
  Calculate Div/4(Out B2) -> Subsystem1/12(Out B2-CD)
  Sign Div result/8(ADD) -> Subsystem1/31(ADD-SDR)
  ALU/5(Overflow) -> Overflow/1
  ALU_REG/1(MOD) -> Sign Div result/3(MOD)
  AND1/1 -> Simulink to PS Bus/1(BusIn)
  DP Read/1 -> AND1/2
  connections:
  Bus Out/RConn1 -- Simulink to PS Bus/RConn1

== system DataPath/Subsystem/ALU ==
  Bus_A : Inport
  Bus_B : Inport  Port=2
  Sel_C : Inport  Port=3
  Sel_B : Inport  Port=4
  Sel_A : Inport  Port=5
  Subtract mode : Inport  Port=6
  SM : Inport  Port=7
  Neg_A : Inport  Port=8
  ALU MUX : Subsystem
      settings: PortSchema="{\"entries\":[{\"content\":{\"sides\":[{\"content\":{\"connectorIds\":[\"In1\",\"In2\",\"In3\",\"In4\",\"In5\",\"In6\",\"In7\",\"In8\",\"In9\",\"In10\",\"In11\",\"In12\",\"In13\",\"In14\",\"In15\",\"In16\"]},\"type\":\"ConnectorPlacement.EquallySpacedRectSide\",\"uuid\":\"e3413fa4-1b2d-4ebe-83ea-8face2a722c4\"},{\"content\":{\"side\":\"RIGHT\"},\"type\":\"ConnectorPlacement.EquallySpacedRectSide\",\"uuid\":\"468a20b8-3e48-40d2-af84-5907293b05d2\"},{\"content\":{\"connectorIds\":[\"Out1\"],\"side\":\"TOP\"},\"type\":\"ConnectorPlacement.EquallySpacedRectSide\",\"uuid\":\"4c8356f8-7f0f-47fd-8d6e-25cf38d6ddc3\"}]},\"type\":\"ConnectorPlacement.EquallySpacedConnector\",\"uuid\":\"84f87871-f62c-4317-8781-2bab8d5e1233\"}],\"packageUris\":[\"http://schema.mathworks.com/mf0/Connector/R2020b\"],\"version\":\"1.0\"}"
  Adder & Logic Module : Subsystem
      settings: PortSchema="{\"entries\":[{\"content\":{\"sides\":[{\"content\":{\"connectorIds\":[\"In1\",\"In2\",\"In3\",\"In4\"]},\"type\":\"ConnectorPlacement.EquallySpacedRectSide\",\"uuid\":\"639aed8e-35a1-4ba0-8b43-3214fbb2c368\"},{\"content\":{\"connectorIds\":[\"Out1\",\"Out2\",\"Out3\",\"Out4\",\"Out5\",\"Out6\",\"Out7\",\"Out8\"],\"side\":\"RIGHT\"},\"type\":\"ConnectorPlacement.EquallySpacedRectSide\",\"uuid\":\"8a439bfb-ce30-47da-a5b4-a54b9d9e640c\"},{\"content\":{\"connectorIds\":[\"Out11\"],\"side\":\"TOP\"},\"type\":\"ConnectorPlacement.EquallySpacedRectSide\",\"uuid\":\"7d81641d-429b-4b81-8cb3-af5c318085c9\"},{\"content\":{\"connectorIds\":[\"Out9\",\"Out10\"],\"side\":\"BOTTOM\"},\"type\":\"ConnectorPlacement.EquallySpacedRectSide\",\"uuid\":\"74152c7b-6851-457b-b5de-2c09c1f82f74\"}]},\"type\":\"ConnectorPlacement.EquallySpacedConnector\",\"uuid\":\"d9b5c2cc-0f19-487b-a2d0-c7259543056d\"}],\"packageUris\":[\"http://schema.mathworks.com/mf0/Connector/R2020b\"],\"version\":\"1.0\"}"
  Delay One Step1 : Delay  DelayLength=1
  Delay One Step3 : Delay  DelayLength=1
  FlagAndDecode : Subsystem
      settings: PortSchema="{\"entries\":[{\"content\":{\"sides\":[{\"content\":{\"connectorIds\":[\"In1\",\"In2\",\"In3\",\"In4\"]},\"type\":\"ConnectorPlacement.EquallySpacedRectSide\",\"uuid\":\"916d1b19-e284-4a28-84cf-bc055bf0c44e\"},{\"content\":{\"connectorIds\":[\"Out1\",\"Out2\",\"Out3\",\"Out4\",\"Out5\",\"Out6\",\"Out7\",\"Out8\"],\"side\":\"RIGHT\"},\"type\":\"ConnectorPlacement.EquallySpacedRectSide\",\"uuid\":\"7130d779-fd13-4a69-b7b9-2dcd4faf046d\"},{\"content\":{\"connectorIds\":[\"Out9\",\"Out10\",\"In5\"],\"side\":\"TOP\"},\"type\":\"ConnectorPlacement.EquallySpacedRectSide\",\"uuid\":\"ce59600e-a31e-4529-9735-bd24f6721c4e\"},{\"content\":{\"connectorIds\":[\"In6\"],\"side\":\"BOTTOM\"},\"type\":\"ConnectorPlacement.EquallySpacedRectSide\",\"uuid\":\"41b3058d-0677-4e1c-be90-f7fc2536099b\"}]},\"type\":\"ConnectorPlacement.EquallySpacedConnector\",\"uuid\":\"b715e1e6-03cb-4b7c-85cc-1984e61b148f\"}],\"packageUris\":[\"http://schema.mathworks.com/mf0/Connector/R2020b\"],\"version\":\"1.0\"}"
  Zero : Outport
  Negative : Outport  Port=2
  A=B : Outport  Port=3
  A>B : Outport  Port=4
  Overflow : Outport  Port=5
  ALU Bus : Outport  Port=6
  wires:
  Subtract mode/1 -> Delay One Step1/1
  Bus_B/1 -> Adder & Logic Module/4(Bus_B)
  Bus_A/1 -> Adder & Logic Module/3(Bus_A)
  Adder & Logic Module/10(A>B) -> A>B/1
  Adder & Logic Module/7(Bus7) -> ALU MUX/15(Bus7)
  Adder & Logic Module/5(Bus5) -> ALU MUX/13(Bus5)
  Adder & Logic Module/3(Bus3) -> ALU MUX/11(Bus3)
  Adder & Logic Module/9(A=B) -> A=B/1
  SM/1 -> FlagAndDecode/1(SM)
  Sel_B/1 -> FlagAndDecode/3(Sel_B)
  Sel_A/1 -> FlagAndDecode/2(Sel_A)
  Sel_C/1 -> FlagAndDecode/4(Sel_C)
  Adder & Logic Module/1(Bus1) -> ALU MUX/9(Bus1)
  Adder & Logic Module/8(Bus8) -> ALU MUX/16(Bus8)
  Adder & Logic Module/6(Bus6) -> ALU MUX/14(Bus6)
  Adder & Logic Module/4(Bus4) -> ALU MUX/12(Bus4)
  Adder & Logic Module/2(Bus2) -> ALU MUX/10(Bus2)
  Adder & Logic Module/11(Overflow) -> Overflow/1, FlagAndDecode/6(Overflow)
  FlagAndDecode/5(1/0/0) -> ALU MUX/5(1/0/0)
  FlagAndDecode/3(0/1/0) -> ALU MUX/3(0/1/0)
  FlagAndDecode/1(0/0/0) -> ALU MUX/1(0/0/0)
  FlagAndDecode/4(0/1/1) -> ALU MUX/4(0/1/1)
  FlagAndDecode/2(0/0/1) -> ALU MUX/2(0/0/1)
  FlagAndDecode/10(Negative) -> Negative/1
  FlagAndDecode/8(1/1/1) -> ALU MUX/8(1/1/1)
  FlagAndDecode/6(1/0/1) -> ALU MUX/6(1/0/1)
  FlagAndDecode/9(Zero) -> Zero/1
  FlagAndDecode/7(1/1/0) -> ALU MUX/7(1/1/0)
  ALU MUX/1(ALU Output) -> FlagAndDecode/5(ALU Bus), ALU Bus/1
  Neg_A/1 -> Delay One Step3/1
  Delay One Step3/1 -> Adder & Logic Module/2(Neg_A)
  Delay One Step1/1 -> Adder & Logic Module/1(Subtract mode)

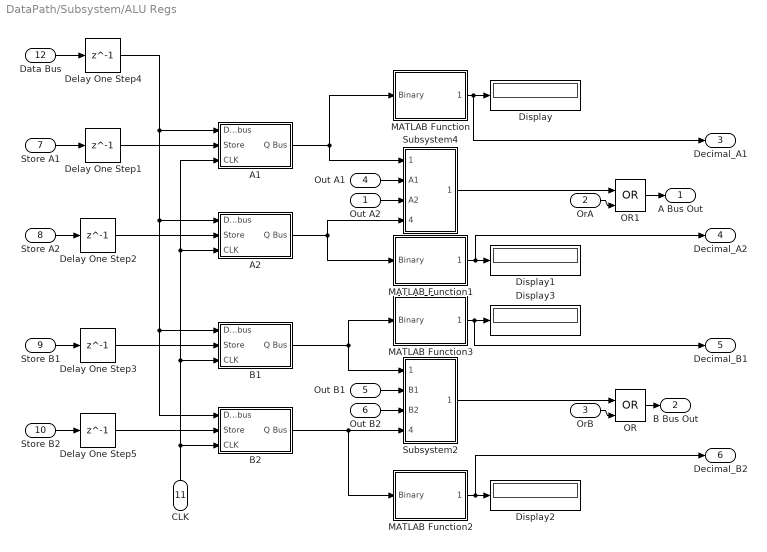
== system DataPath/Subsystem/ALU Regs ==
  Out A2 : Inport
  OrA : Inport  Port=2
  OrB : Inport  Port=3
  Out A1 : Inport  Port=4
  Out B1 : Inport  Port=5
  Out B2 : Inport  Port=6
  Store A1 : Inport  Port=7
  Store A2 : Inport  Port=8
  Store B1 : Inport  Port=9
  Store B2 : Inport  Port=10
  CLK : Inport  Port=11
  Data Bus : Inport  Port=12
  A1 : Subsystem
  A2 : Subsystem
  B1 : Subsystem
  B2 : Subsystem
  Delay One Step{1..5} (5 alike) : Delay  DelayLength=1
  Display{,1..3} (4 alike) : Display
  MATLAB Function : MATLAB Function  TreatAsAtomicUnit=on
  MATLAB Function1 : MATLAB Function  TreatAsAtomicUnit=on
  MATLAB Function2 : MATLAB Function  TreatAsAtomicUnit=on
  MATLAB Function3 : MATLAB Function  TreatAsAtomicUnit=on
  OR : Logic  Operator=OR  IconShape=distinctive  AllPortsSameDT=off  OutDataTypeStr=boolean
  OR1 : Logic  Operator=OR  IconShape=distinctive  AllPortsSameDT=off  OutDataTypeStr=boolean
  Subsystem2 : Subsystem
  Subsystem4 : Subsystem
  A Bus Out : Outport
  B Bus Out : Outport  Port=2
  Decimal_A1 : Outport  Port=3
  Decimal_A2 : Outport  Port=4
  Decimal_B1 : Outport  Port=5
  Decimal_B2 : Outport  Port=6
  wires:
  CLK/1 -> A1/3(CLK), A2/3(CLK), B1/3(CLK), B2/3(CLK)
  Data Bus/1 -> Delay One Step4/1
  Out A1/1 -> Subsystem4/2(A1)
  Out A2/1 -> Subsystem4/3(A2)
  Store B1/1 -> Delay One Step3/1
  Out B1/1 -> Subsystem2/2(B1)
  Store B2/1 -> Delay One Step5/1
  Subsystem4/1(But Out) -> OR1/1
  Subsystem2/1(But Out) -> OR/1
  MATLAB Function2/1(Decimal) -> Decimal_B2/1, Display2/1
  MATLAB Function1/1(Decimal) -> Decimal_A2/1, Display1/1
  B1/1("Q Bus ") -> Subsystem2/1(Bus B1), MATLAB Function3/1(Binary)
  B2/1("Q Bus ") -> MATLAB Function2/1(Binary), Subsystem2/4(Bus B 2)
  A1/1("Q Bus ") -> Subsystem4/1(Bus A1), MATLAB Function/1(Binary)
  MATLAB Function3/1(Decimal) -> Decimal_B1/1, Display3/1
  A2/1("Q Bus ") -> MATLAB Function1/1(Binary), Subsystem4/4(Bus A2)
  MATLAB Function/1(Decimal) -> Decimal_A1/1, Display/1
  Out B2/1 -> Subsystem2/3(B2)
  Store A2/1 -> Delay One Step2/1
  Store A1/1 -> Delay One Step1/1
  OR/1 -> B Bus Out/1
  OR1/1 -> A Bus Out/1
  OrA/1 -> OR1/2
  OrB/1 -> OR/2
  Delay One Step4/1 -> A1/1(Data bus), A2/1(Data bus), B1/1(Data bus), B2/1(Data bus)
  Delay One Step1/1 -> A1/2(Store)
  Delay One Step2/1 -> A2/2(Store)
  Delay One Step3/1 -> B1/2(Store)
  Delay One Step5/1 -> B2/2(Store)

== system DataPath/Subsystem/ALU_REG ==
  Data bus : Inport
  Store : Inport  Port=2
  CLK : Inport  Port=3
  Demux : Demux  Outputs=8
  Subsystem1 : Subsystem
  Subsystem3 : Subsystem
  MOD : Outport
  SM : Outport  Port=2
  wires:
  Data bus/1 -> Demux/1
  Store/1 -> Subsystem1/2(Store), Subsystem3/2(Store)
  CLK/1 -> Subsystem1/3(Clock), Subsystem3/3(Clock)
  Subsystem3/1(Q) -> MOD/1
  Subsystem1/1(Q) -> SM/1
  Demux/7 -> Subsystem3/1(Data)
  Demux/8 -> Subsystem1/1(Data)

== system DataPath/Subsystem/Add Subtract Logic ==
  Shift Right : Inport
  Shift Left : Inport  Port=2
  AND : Inport  Port=3
  OR : Inport  Port=4
  XOR : Inport  Port=5
  NOT A : Inport  Port=6
  NOT B : Inport  Port=7
  Subtract : Inport  Port=8
  Evaluate : Inport  Port=9
  Operation : Inport  Port=10
  Add : Inport  Port=11
  LO : Inport  Port=12
  AND2 : Logic  IconShape=distinctive  AllPortsSameDT=off  OutDataTypeStr=boolean
  OR14 : Logic  Operator=OR  Inputs=3  IconShape=distinctive  AllPortsSameDT=off  OutDataTypeStr=boolean
  Subsystem1 : Subsystem
  Subsystem2 : Subsystem
  ALU,DP,A1,B1 : Outport
  C Stored : Outport  Port=2
  B Stored : Outport  Port=3
  A Stored : Outport  Port=4
  wires:
  Shift Right/1 -> Subsystem1/6(SR)
  Shift Left/1 -> Subsystem1/7(SL)
  AND/1 -> Subsystem1/1(AND)
  XOR/1 -> Subsystem1/3(XOR)
  OR/1 -> Subsystem1/2(OR)
  NOT A/1 -> Subsystem1/4(!A)
  NOT B/1 -> Subsystem1/5("!B ")
  Subtract/1 -> OR14/2
  Add/1 -> OR14/1
  Operation/1 -> Subsystem2/2(Enable)
  Subsystem2/1(A Stored) -> A Stored/1
  LO/1 -> OR14/3, Subsystem2/1(LO)
  OR14/1 -> AND2/2
  Evaluate/1 -> AND2/1
  Subsystem2/3(C Stored) -> C Stored/1
  Subsystem2/2(B Stored) -> B Stored/1
  AND2/1 -> ALU,DP,A1,B1/1
  Subsystem1/1(C) -> Subsystem2/3(C)
  Subsystem1/2(B) -> Subsystem2/4(B)
  Subsystem1/3("A ") -> Subsystem2/5(A)

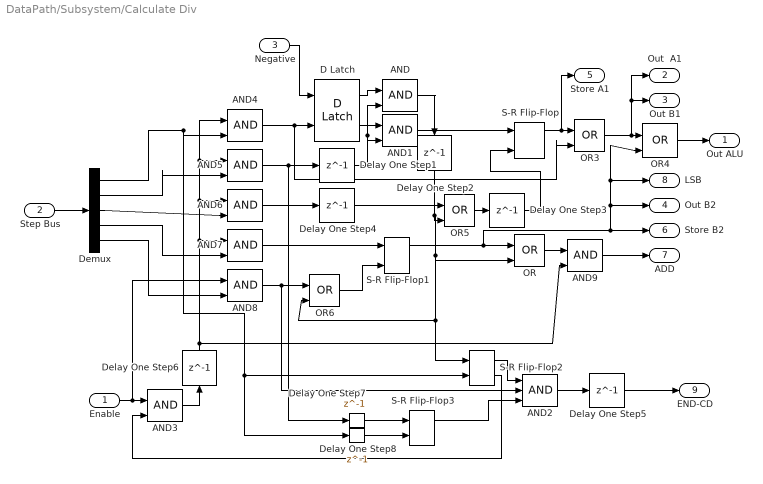
== system DataPath/Subsystem/Calculate Div ==
  Enable : Inport
  Step Bus : Inport  Port=2
  Negative : Inport  Port=3
  AND{,1,3..9} (9 alike) : Logic  IconShape=distinctive  AllPortsSameDT=off  OutDataTypeStr=boolean
  AND2 : Logic  Inputs=3  IconShape=distinctive  AllPortsSameDT=off  OutDataTypeStr=boolean
  D Latch : simulink_extras/Flip Flops/D Latch
  Delay One Step{1..6} (6 alike) : Delay  DelayLength=1
  Delay One Step7 : Delay  DelayLength=1  SampleTime=1e-6
  Delay One Step8 : Delay  DelayLength=1  SampleTime=1e-6
  Demux : Demux  Outputs=5
  OR{,3..6} (5 alike) : Logic  Operator=OR  IconShape=distinctive  AllPortsSameDT=off  OutDataTypeStr=boolean
  S-R Flip-Flop{,1..3} (4 alike) : simulink_extras/Flip Flops/S-R Flip-Flop  initial_condition=0
  Out ALU : Outport
  Out  A1 : Outport  Port=2
  Out B1 : Outport  Port=3
  Out B2 : Outport  Port=4
  Store A1 : Outport  Port=5
  Store B2 : Outport  Port=6
  ADD : Outport  Port=7
  LSB : Outport  Port=8
  END-CD : Outport  Port=9
  wires:
  Step Bus/1 -> Demux/1
  Demux/4 -> AND7/2
  Demux/1 -> Delay One Step8/1, S-R Flip-Flop2/2, AND4/2
  Demux/3 -> AND6/2
  Demux/2 -> AND5/2
  AND3/1 -> Delay One Step6/1
  Demux/5 -> AND8/2
  OR/1 -> AND9/1
  AND9/1 -> ADD/1
  Negative/1 -> D Latch/1
  D Latch/1 -> AND/1
  D Latch/2 -> AND1/1
  AND1/1 -> S-R Flip-Flop/1
  OR4/1 -> Out ALU/1
  OR3/1 -> Out B1/1, Out  A1/1, OR4/1
  Delay One Step3/1 -> S-R Flip-Flop/2
  S-R Flip-Flop1/1 -> Out B2/1, OR4/2, LSB/1, Store B2/1, OR/1
  AND4/1 -> OR3/2, D Latch/2
  AND5/1 -> Delay One Step7/1, Delay One Step1/1
  AND6/1 -> Delay One Step4/1
  OR6/1 -> S-R Flip-Flop1/2
  AND7/1 -> S-R Flip-Flop1/1
  AND8/1 -> AND2/2, OR6/1
  S-R Flip-Flop/1 -> Store A1/1, OR3/1
  AND/1 -> Delay One Step2/1
  S-R Flip-Flop2/1 -> AND2/1
  AND2/1 -> Delay One Step5/1
  Enable/1 -> AND8/1, AND3/1
  S-R Flip-Flop2/2 -> AND3/2
  Delay One Step4/1 -> OR5/1
  OR5/1 -> Delay One Step3/1
  Delay One Step1/1 -> AND/2, AND1/2
  Delay One Step2/1 -> S-R Flip-Flop2/1, OR6/2, OR/2, OR5/2
  Delay One Step5/1 -> END-CD/1
  Delay One Step6/1 -> AND4/1, AND5/1, AND6/1, AND7/1, AND9/2
  S-R Flip-Flop3/1 -> AND2/3
  Delay One Step7/1 -> S-R Flip-Flop3/1
  Delay One Step8/1 -> S-R Flip-Flop3/2

== system DataPath/Subsystem/DP PORT ==
  note: Real System will use a TSB not and Gates
  DP Bus : Inport
  Enable : Inport  Port=2
  AND{7..14} (8 alike) : Logic  IconShape=distinctive  AllPortsSameDT=off  OutDataTypeStr=boolean
  Demux : Demux  Outputs=8
  Mux : Mux  Inputs=8
  DP Output : Outport
  wires:
  Demux/3 -> AND9/1
  Enable/1 -> AND7/2, AND8/2, AND9/2, AND10/2, AND12/2, AND13/2, AND14/2, AND11/2
  Demux/4 -> AND10/1
  Demux/1 -> AND7/1
  AND12/1 -> Mux/5
  Demux/8 -> AND11/1
  Demux/6 -> AND13/1
  AND14/1 -> Mux/7
  Demux/2 -> AND8/1
  AND13/1 -> Mux/6
  Demux/7 -> AND14/1
  AND9/1 -> Mux/3
  DP Bus/1 -> Demux/1
  AND7/1 -> Mux/1
  AND10/1 -> Mux/4
  Demux/5 -> AND12/1
  AND8/1 -> Mux/2
  AND11/1 -> Mux/8
  Mux/1 -> DP Output/1
